simulink model "untitled"  (R2019a)
settings: Solver=VariableStepAuto  StartTime=0.0  StopTime=10.0  RelTol=1e-3
settings Model: Creator=ananya  LastModifiedBy=ananya

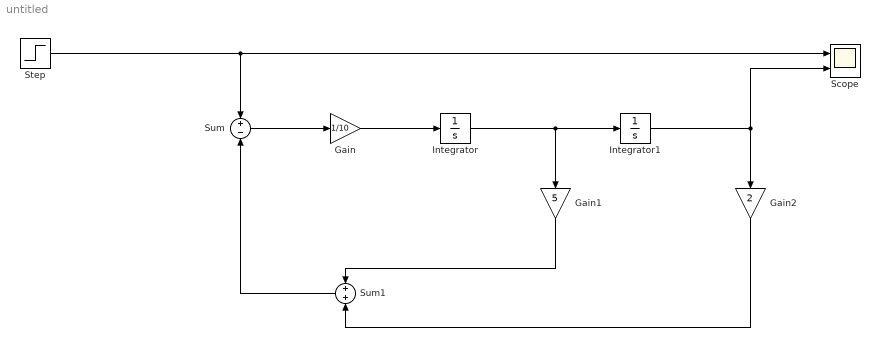
== system untitled ==
  Gain : Gain  Gain=1/10
  Gain1 : Gain  Gain=5
  Gain2 : Gain  Gain=2
  Integrator : Integrator
  Integrator1 : Integrator
  Scope : Scope  NumInputPorts=2
  Step : Step  SampleTime=0
  Sum : Sum  Inputs=+-
  Sum1 : Sum
  wires:
  Sum/1 -> Gain/1
  Gain/1 -> Integrator/1
  Integrator/1 -> Gain1/1, Integrator1/1
  Sum1/1 -> Sum/2
  Step/1 -> Scope/1, Sum/1
  Integrator1/1 -> Gain2/1, Scope/2
  Gain2/1 -> Sum1/2
  Gain1/1 -> Sum1/1
